simulink model "j4SimTestBench"  (R2016b)
settings: Solver=VariableStepAuto  StartTime=0.0  StopTime=100  RelTol=1e-3
undefined symbols (not defined in the file or in its folder): filtNum
libraries: simulink x2, dcpctrl x2, dsparch4 x1
settings Model: Creator=julianleland  LastModifiedBy=julianleland

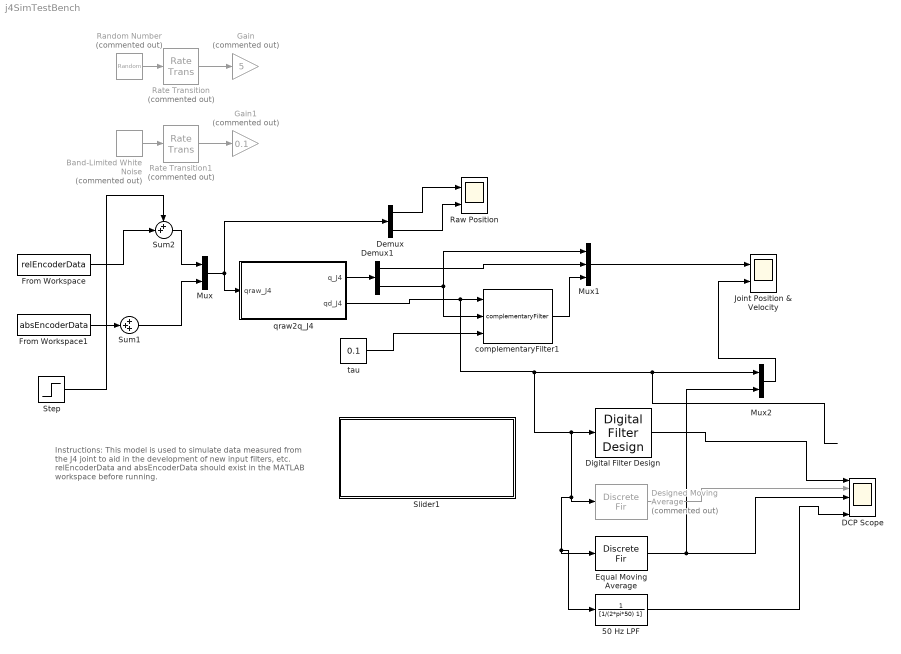
== system j4SimTestBench ==
  note: Instructions:
      |
      | This model is used to simulate data measured from the J4 joint to aid in the development of new input filters, etc. relEncoderData and absEncoderData should exist in the MATLAB workspace before running.
  50 Hz LPF : TransferFcn  Denominator=[1/(2*pi*50) 1]
  Band-Limited White Noise : simulink/Sources/Band-Limited White Noise  Commented=on  Cov=[0.1]  Ts=0.01  seed=[23341]
  DCP Scope : Scope  NumInputPorts=5
  Demux : Demux  Outputs=2
  Demux1 : Demux  Outputs=2
  Designed Moving Average : DiscreteFir  Commented=on  Coefficients=filtNum  InputProcessing=Columns as channels (frame based)
  Digital Filter Design : dsparch4/Digital Filter Design  mwdsp_browser_bugfix_var=off
  Equal Moving Average : DiscreteFir  Coefficients=repmat([1/20],1,20)  InputProcessing=Columns as channels (frame based)
  From Workspace : FromWorkspace  VariableName=relEncoderData  OutDataTypeStr=double  SampleTime=.001  Interpolate=off  OutputAfterFinalValue=Holding final value
  From Workspace1 : FromWorkspace  VariableName=absEncoderData  SampleTime=.001  Interpolate=off  OutputAfterFinalValue=Holding final value
  Gain : Gain  Commented=on  Gain=5
  Gain1 : Gain  Commented=on  Gain=0.1
  Joint Position & Velocity : Scope  NumInputPorts=2
  Mux : Mux  Inputs=2
  Mux1 : Mux  Inputs=3
  Mux2 : Mux  Inputs=2
  Random Number : RandomNumber  Commented=on  SampleTime=10
  Rate Transition : RateTransition  Commented=on
  Rate Transition1 : RateTransition  Commented=on
  Raw Position : Scope  NumInputPorts=2
  Slider1 : Subsystem  DialogController=hmiCreateDDGDialog  IsWebBlock=on  mask(MWDashboardBlock){webBlockId=31488d2d-c555-48c9-95df-eb45209c2152, webBlockType=slider, ShowInLibBrowser=on, ShowInitialText=on, HMISrcModelName=j4SimTestBench}
      mask prompts: webBlockId "WebBlock Id"; webBlockType "WebBlock Type"; HMISrcModelName "Source Model"
      mask help: SimulinkHMI:dialogs:SliderDialogDesc
      mask Help: helpview([docroot '/mapfiles/simulink.map'], 'hmi_slider')
      mask Display:
      | if strcmp(get_param(bdroot(gcb),'BlockDiagramType'), 'library')
      |     image([(matlabroot) '/toolbox/simulink/hmi/icons/Slider.png']);
      | end
  Step : Step  Time=40  After=10000
  Sum1 : Sum  Inputs=+++
  Sum2 : Sum  Inputs=++|
  complementaryFilter1 : dcpctrl/complementaryFilter
  qraw2q_J4 : Subsystem
  tau : Constant  Value=0.1
  wires:
  Sum2/1 -> Mux/1
  Sum1/1 -> Mux/2
  Demux/1 -> Raw Position/1
  Demux/2 -> Raw Position/2
  Mux/1 -> qraw2q_J4/1(qraw_J4), Demux/1
  qraw2q_J4/1(q_J4) -> Demux1/1
  tau/1 -> complementaryFilter1/3
  qraw2q_J4/2(qd_J4) -> 50 Hz LPF/1, Equal Moving Average/1, Designed Moving Average/1, Digital Filter Design/1, Mux2/1, complementaryFilter1/1
  Demux1/1 -> Mux1/2
  complementaryFilter1/1 -> Mux1/3
  Mux1/1 -> Joint Position & Velocity/1
  Band-Limited White Noise/1 -> Rate Transition1/1
  Rate Transition1/1 -> Gain1/1
  Demux1/2 -> Mux1/1, complementaryFilter1/2
  Random Number/1 -> Rate Transition/1
  Rate Transition/1 -> Gain/1
  From Workspace/1 -> Sum2/2
  From Workspace1/1 -> Sum1/2
  Mux2/1 -> Joint Position & Velocity/2
  Digital Filter Design/1 -> DCP Scope/1
  Equal Moving Average/1 -> Mux2/2, DCP Scope/3
  50 Hz LPF/1 -> DCP Scope/5
  Designed Moving Average/1 -> DCP Scope/2
  Step/1 -> Sum2/1

== system j4SimTestBench/Slider1 ==

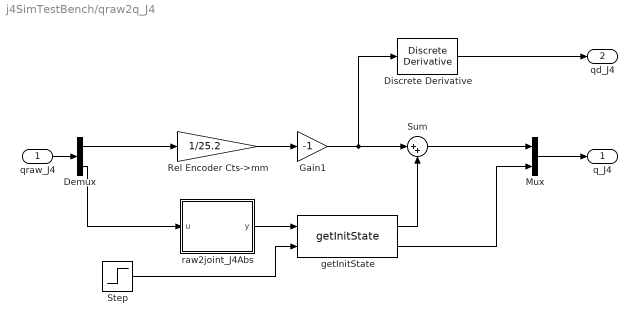
== system j4SimTestBench/qraw2q_J4 ==
  qraw_J4 : Inport
  Demux : Demux  Outputs=2
  Discrete Derivative : simulink/Discrete/Discrete Derivative  gainval=1.0  ICPrevScaledInput=0.0  OutMin=[]  OutMax=[]  OutDataType=fixdt(1, 16)  OutScaling=2^-10  DoSatur=off
  Gain1 : Gain  Gain=-1
  Mux : Mux  Inputs=2
  Rel Encoder Cts->mm : Gain  Gain=1/25.2
  Step : Step  Time=0  SampleTime=0
  Sum : Sum  Inputs=|++
  getInitState : dcpctrl/getInitState
  raw2joint_J4Abs : MATLAB Function  TreatAsAtomicUnit=on
  q_J4 : Outport
  qd_J4 : Outport  Port=2
  wires:
  raw2joint_J4Abs/1(y) -> getInitState/1
  Mux/1 -> q_J4/1
  getInitState/2 -> Mux/2
  qraw_J4/1 -> Demux/1
  Demux/2 -> raw2joint_J4Abs/1(u)
  getInitState/1 -> Sum/2
  Step/1 -> getInitState/2
  Demux/1 -> Rel Encoder Cts->mm/1
  Rel Encoder Cts->mm/1 -> Gain1/1
  Sum/1 -> Mux/1
  Discrete Derivative/1 -> qd_J4/1
  Gain1/1 -> Discrete Derivative/1, Sum/1

== matlab function j4SimTestBench/qraw2q_J4/raw2joint_J4Abs ==
  data: u input; y output; robot parameter
function y = fcn(u,robot)

%#codegen

y_temp = raw2jointJ4Abs_at40gw(robot,u');
y = y_temp';
